simulink model "butterworth_test_model"  (R2012b)
settings: Solver=VariableStepDiscrete  StartTime=0.0  StopTime=10.0  RelTol=1e-3
settings Model: Creator=Tomasz  LastModifiedBy=Tomasz

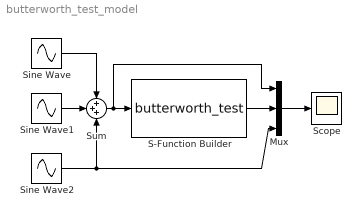
== system butterworth_test_model ==
  Mux : Mux  Inputs=3
  S-Function Builder : S-Function  InitFcn=try, set_param(gcb,'FunctionName','butterworth_test'), end  FunctionName=butterworth_test  SFunctionModules=butterworth_test_wrapper butterworth  EnableBusSupport=off  mask(S-Function Builder){}
      mask help: Simulink:masks:SFunctionBuilder_MD
      mask init:
      | val = [[.9  0.75 0.75 1 1 .9 .9 1]',[1 1 0.75 0.75 .9 .9 1 .9]'];try , sys = get_param(gcb,'SfunBuilderFcnName');if isempty(sys), sys = get_param(gcb,'FunctionName'); end,catch, sys = get_param(gcb,'FunctionName'); end
      settings: CopyFcn=set_param(gcbh,'LinkStatus','none')  PreSaveFcn=try, set_param(gcb,'FunctionName','butterworth_test'), end  OpenFcn=sfunctionwizard(gcbh)
      mask Display: plot(val(:,1),val(:,2)),disp(sys), port_label('input',1,'u0'), port_label('output',1,'y0')
  Scope : Scope
      settings: TickLabels=on  TimeRange=1  YMin=-2.5  YMax=2.5  MaxDataPoints=10e4
  Sine Wave : Sin  Frequency=250 * 2*pi  Phase=30 / 180 * pi  SampleTime=1e-4
  Sine Wave1 : Sin  Frequency=150 * 2*pi  Phase=10 / 180 * pi  SampleTime=1e-4
  Sine Wave2 : Sin  Frequency=50 * 2*pi  Phase=5 / 180 * pi  SampleTime=1e-4
  Sum : Sum  Inputs=+++
  wires:
  Sine Wave/1 -> Sum/1
  Sine Wave1/1 -> Sum/2
  Sine Wave2/1 -> Mux/3, Sum/3
  Sum/1 -> Mux/1, S-Function Builder/1
  Mux/1 -> Scope/1
  S-Function Builder/1 -> Mux/2
